simulink model "alignment_bending_procedure_n_6"  (R2018b)
settings: Solver=VariableStepAuto  StartTime=0.0  StopTime=6  RelTol=1e-3
values from neighbouring files (symbols this model uses):
  base_size = [0.2 0.3 1.5]    [robot_setup.m]    (also in robot_setup_bis.m)
  beam_length = 1.14    [robot_setup.m]    (also in robot_setup_bis.m)
  beam_radius = 0.032    [robot_setup.m]    (also in robot_setup_bis.m)
  beam_state_wf_des = fixture_keypoints(fixture_height, fixture_y, n_keypoints)    [robot_setup.m]    (also in robot_setup_bis.m)
  fixture_height = 1.5    [robot_setup.m]    (also in robot_setup_bis.m)
  fixture_x = 0.8    [robot_setup.m]    (also in robot_setup_bis.m)
  J = fscanf(fileID, '    [jacobian_mean_std.m]    (also in robot_setup.m = J_array{i-n_start+1}; robot_setup_bis.m = J_array{i-n_start+1})
  n_keypoints = i    [robot_setup.m]    (also in robot_setup_bis.m)
  robot_frame_x = 0.15    [robot_setup.m]    (also in robot_setup_bis.m)
  T = 0.005    [robot_setup.m]    (also in robot_setup_bis.m; sim_robot_control_error.m)
  wf_T_rf_left = [R_left, xyz_left'; 0 0 0 1]    [robot_setup.m]    (also in robot_setup_bis.m)
  wf_T_rf_right = [R_right, xyz_right'; 0 0 0 1]    [robot_setup.m]    (also in robot_setup_bis.m)
  xyz_0_rf_left = xyz_0_rf_left(1:3)    [robot_setup.m]    (also in robot_setup_bis.m)
  xyz_0_rf_right = xyz_0_rf_right(1:3)    [robot_setup.m]    (also in robot_setup_bis.m)
undefined symbols (not defined in the file or in its folder): beam_wall, beam_width, Extr_Data_Box, Levenberg, Marquardt, X, Y, Z
libraries: sm_lib x331, nesl_utility x53, sm_flex_body_lib x12, robotcorelib x4, simulink x2, robotmaniplib x2
(part 1 of 8)
settings Model: Creator=alberto  LastModifiedBy=alberto

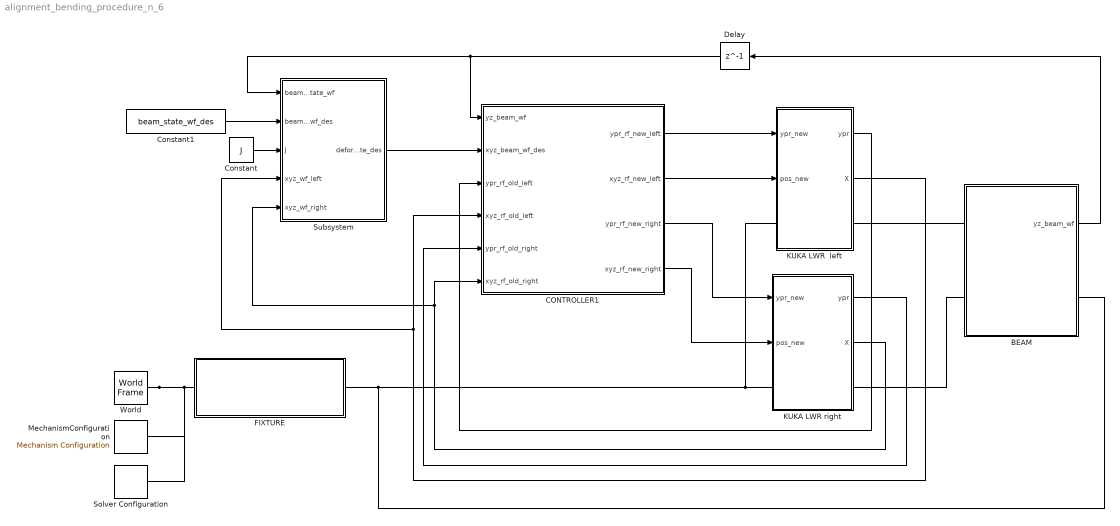
== system alignment_bending_procedure_n_6 ==
  BEAM : Subsystem
  CONTROLLER1 : Subsystem
  Constant : Constant  Value=J
  Constant1 : Constant  Value=beam_state_wf_des
  Delay : Delay  DelayLength=1  InitialCondition=-9999*ones(2*n_keypoints,1)
  FIXTURE : Subsystem
  KUKA LWR  left : Subsystem  mask{base_initial_position=[0 robot_frame_x base_size(3)-0.1]', base_initial_orientation=[pi/2 0 -pi/2]', ee_initial_position=xyz_0_rf_left, ee_initial_orientation=[0 5*pi/6 0]'}
      mask prompts: base_initial_position "base initial position [x y z]' (m)"; base_initial_orientation "base initial orientation [y p r]' (rad)"; ee_initial_position "ee initial position [x y z]' (m)"; ee_initial_orientation "ee initial orientation [y p r]' (rad)"
  KUKA LWR right : Subsystem  mask{base_initial_position=[0 -robot_frame_x base_size(3)-0.1]', base_initial_orientation=[-pi/2 0 pi/2]', ee_initial_position=xyz_0_rf_right, ee_initial_orientation=[0 5*pi/6 0]'}
      mask prompts: base_initial_position "base initial position [x y z]' (m)"; base_initial_orientation "base initial orientation [y p r]' (rad)"; ee_initial_position "ee initial position [x y z]' (m)"; ee_initial_orientation "ee initial orientation [y p r]' (rad)"
  MechanismConfiguration : sm_lib/Utilities/Mechanism Configuration  UniformGravity=Constant  GravityVector=[0 0 -9.80665]  GravityUnits=m/s^2  LinearizationDelta=0.001
  Solver Configuration : nesl_utility/Solver Configuration  PhysicalDomain=network_engine_domain  SubClassName=solver  LeftPortType=input  RightPortType=generic  Tones=[]  Harmonics=[]  SimulateNoise=off  Profile=off  UseLocalSampling=off  EnableSwitchedLinearOptims=on  FrequencyDomain=off  UseCCode=off  RelTol=0.001  AbsTol=1e-06  MinStep=1e-09  ToWorkspace=off  RevertToSquareIcSolve=off  NumHomotopyIterations=100  PhasorMode=off  PhasorModeNumHarmonics=1  DoDC=off  ResidualTolerance=1e-09  UseLocalSolver=off  LocalSolverChoice=NE_BACKWARD_EULER_ADVANCER  LocalSolverSampleTime=0.001  DoFixedCost=off  MaxNonlinIter=3  MaxModeIter=2  LinearAlgebra=auto  EquationFormulation=NE_TIME_EF  DelaysMemoryBudget=1024  AutomaticFiltering=on  FilteringTimeConstant=0.001  PartitionStorageMethod=AS_NEEDED  PartitionMemoryBudget=1024
  Subsystem : Subsystem
  World : sm_lib/Frames and Transforms/World Frame
  wires:
  KUKA LWR right/1(ypr) -> CONTROLLER1/5(ypr_rf_old_right)
  CONTROLLER1/1(ypr_rf_new_left) -> KUKA LWR  left/1(ypr_new)
  KUKA LWR  left/1(ypr) -> CONTROLLER1/3(ypr_rf_old_left)
  KUKA LWR  left/2(X) -> CONTROLLER1/4(xyz_rf_old_left), Subsystem/4(xyz_wf_left)
  CONTROLLER1/2(xyz_rf_new_left) -> KUKA LWR  left/2(pos_new)
  KUKA LWR right/2(X) -> CONTROLLER1/6(xyz_rf_old_right), Subsystem/5(xyz_wf_right)
  CONTROLLER1/4(xyz_rf_new_right) -> KUKA LWR right/2(pos_new)
  CONTROLLER1/3(ypr_rf_new_right) -> KUKA LWR right/1(ypr_new)
  Constant1/1 -> Subsystem/2(beam_state_wf_des)
  Constant/1 -> Subsystem/3(J)
  Subsystem/1(deformation_state_des) -> CONTROLLER1/2(xyz_beam_wf_des)
  Delay/1 -> CONTROLLER1/1(yz_beam_wf), Subsystem/1(beam_state_wf)
  BEAM/1("yz_beam_wf ") -> Delay/1
  connections:
  BEAM/LConn1 -- KUKA LWR  left/RConn1
  KUKA LWR  left/LConn1 -- BEAM/RConn1 -- FIXTURE/RConn1 -- KUKA LWR right/LConn1
  BEAM/LConn2 -- KUKA LWR right/RConn1
  World/RConn1 -- Solver Configuration/RConn1 -- MechanismConfiguration/RConn1 -- FIXTURE/LConn1

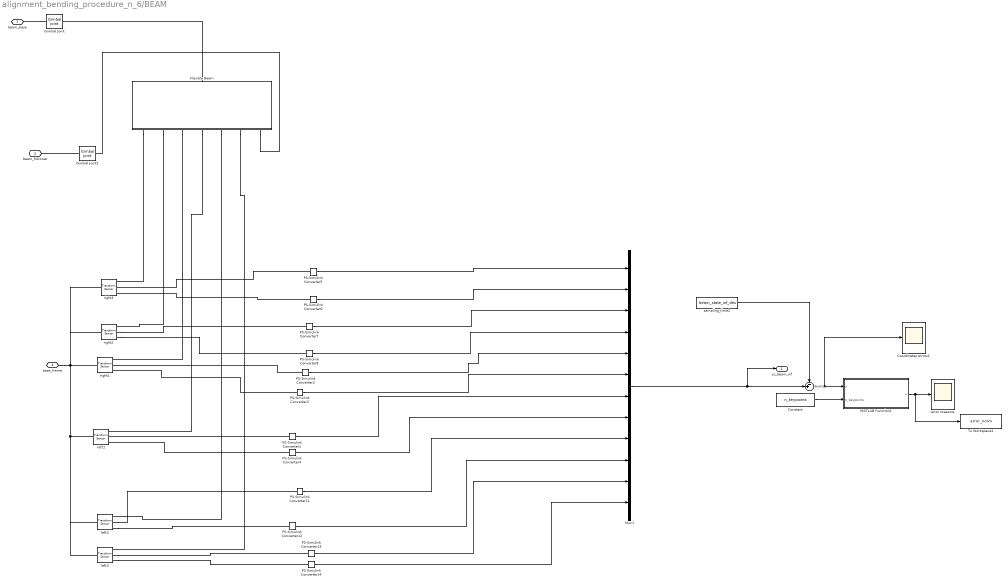
== system alignment_bending_procedure_n_6/BEAM ==
  Constant : Constant  Value=n_keypoints
  Coordinates errors1 : Scope
  Flexible Beam : Subsystem  Tag=PublishSubsystem  AncestorBlock=sm_flex_body_lib/Lumped Parameter/Bodies/Flexible Beam  mask(Flexible Body, Lumped Parameter){popup_material=Aluminum, rho_cust=975, youngsM_cust=0.8e+9, shearM_cust=0.117e+9, rho_std=2.800e+03, youngsM_std=7.000e+10, shearM_std=2.700e+10, edf_beam=2.5807e-05, sdf_beam=3.2259e-06, checkbox_internalvalues=off, popup_xc=Hollow Circle, beam_width=0.05, beam_width_in=0, beam_height=0.005, beam_height_in=0, circle_diameter=beam_radius, circle_diameter_in=0, custom_ixx=2.6121e-003, custom_iyy=2.6121e-003, custom_ip=5.2242e-003, custom_j=1.5625e-09, extrusion_data_custom=[0.015 0.005;-0.015 0.005;-0.015 -0.005;0.015 -0.005]/2, beam_length=beam_length, elem_length=0.095, numelem=12, extrusion_data=Extr_Data_Box(beam_width,beam_width-2*beam_wall,beam_width,beam_width-2*beam_wall), beam_color=[0 1 0], beam_opacity=1, radio_flextype=Rotation: Z}
      mask prompts: checkbox_internalvalues "Print internal values to Command Window"; popup_xc "Cross-Section Type"; custom_ixx "Area Ixx"; custom_iyy "Area Iyy"; custom_ip "Polar Ip"; custom_j "Torsion J (m^4)"; extrusion_data_custom "Extrusion data [x;y] (m)"; beam_length "Length (m)"; numelem "Number of elements"; beam_color "Color [RGB]"; beam_opacity "Opacity (0-1)"; radio_flextype "Flexible Element Degrees of Freedom"
      mask help: Models a flexible beam based on lumped parameter method. Number of flexible elements, material properties as well as beam cross section and dimensions can be varied from mask parameters.
      mask init:
      | cur_blk = gcb;
      | 
      | if(popup_xc==1)
      |     extrusion_data = Extr_Data_Box(beam_width,beam_width_in,beam_height,beam_height_in);
      |     xc_props = [beam_width beam_width_in beam_height beam_height_in];
      | elseif(popup_xc==2)
      |     extrusion_data = Extr_Data_Ring(circle_diameter/2,circle_diameter_in/2,0,360);
      |     xc_props = [circle_diameter circle_diameter_in];
      | elseif(popup_xc==3)
      |     extrusion_data = extrusion_data_custom;
      |     extrusion_data_vec = reshape(extrusion_data,[length(extrusion_data)*2,1]);
      |     xc_props = [custom_ixx;custom_iyy;custom_ip;custom_j;extrusion_data_vec];
      | end
      | 
      | if(popup_material == 1)
      |     rho = rho_cust;
      |     youngsM = youngsM_cust;
      |     shearM = shearM_cust;
      | else
      |     rho = rho_std;
      |     youngsM = youngsM_std;
      |     shearM = shearM_std;
      | end
      | 
      | 
      | [krot_beamz, krot_beamy, krot_beamx, ktra_beamx,...
      |     brot_beamz, brot_beamy, brot_beamx, btra_beamx, ...
      |     elem_length, Ixx, Iyy, J, crossArea] = ...
      |     sm_flex_body_lib_lpar_compute_flexprop(youngsM, shearM, numelem, beam_length, ...
      |     edf_beam, sdf_beam,popup_xc, xc_props);
      | 
      | if(checkbox_internalvalues)
      |     temp_intvaltable = table(...
      |         [Ixx;Iyy;J;crossArea;elem_length;...
      |         krot_beamz;krot_beamy;krot_beamx;ktra_beamx;...
      |         brot_beamz;brot_beamy;brot_beamx;btra_beamx],...
      |         {'m^4';'m^4';'m^4';'m^2';'m';...
      |         'N*m/rad';'N*m/rad';'N*m/rad';'N/m';...
      |         'N*m/(rad/s)';'N*m/(rad/s)';'N*m/(rad/s)';'N/(m/s)'},...
      |         'VariableNames',{'Value','Units'},'RowNames',...
      |         {'Area Moment of Inertia, Ixx','Area Moment of Inertia, Iyy',...
      |         'Torsional Constant, J','Cross sectional area, A','Flexible element length',...
      |         'Element Stiffness, Bending about Z','Element Stiffness, Bending about Y',...
      |         'Element Stiffness, Torsion about X','Element Stiffness, Elongation along X',...
      |         'Element Damping, Bending about Z','Element Damping, Bending about Y',...
      |         'Element Damping, Torsion about X','Element Damping, Elongation along X'});
      |     disp(temp_intvaltable);
      | end
      | 
      | set_param(cur_blk,'elem_length',num2str(elem_length));
      | 
      | sm_flex_body_lib_lpar_construct_beam(cur_blk,numelem,get_param(cur_blk,'radio_flextype'));
      | 
      | clear xc_props
      settings: CopyFcn=%set_param(gcb, 'LinkStatus', 'none')
      settings: AttributesFormatString=|
      | No of Elem: 12
      | Rotation: Z
      mask Help: web('sm_flex_body_lib_lumped_par_beam.html')
      mask TypeOptions popup_material: Custom | Steel | Aluminum | Brass | Bismuth | Copper | Gold | Iron | Lead | Magnesium | Nickel | Silver | Tin | Zinc
      mask Callback popup_material:
      | maskObj = Simulink.Mask.get(gcb);
      | contcm_h = maskObj.getDialogControl('cont_custmaterial');
      | contsm_h = maskObj.getDialogControl('cont_stdmaterial');
      | 
      | rhostd_h = maskObj.getParameter('rho_std');
      | youngM_h = maskObj.getParameter('youngsM_std');
      | shearM_h = maskObj.getParameter('shearM_std');
      | 
      | popup_cm = get_param(gcb,'popup_material');
      | if strcmp(popup_cm,'Custom')
      |     contcm_h.Visible = 'on';
      |     contsm_h.Visible = 'off';
      | else
      |     [rho, E, G] = sm_flex_body_lib_lpar_matprops(popup_cm);
      |     rhostd_h.ReadOnly = 'off';
      |     youngM_h.ReadOnly = 'off';
      |     shearM_h.ReadOnly = 'off';
      |     set_param(gcb,'rho_std',sprintf('%0.3e',rho));
      |     set_param(gcb,'youngsM_std',sprintf('%0.3e',E));
      |     set_param(gcb,'shearM_std',sprintf('%0.3e',G));
      | 	rhostd_h.ReadOnly = 'on';
      |     youngM_h.ReadOnly = 'on';
      |     shearM_h.ReadOnly = 'on';
      |     contcm_h.Visible = 'off';
      |     contsm_h.Visible = 'on';
      | end
      | 
      | clear maskObj contcm_h contsm_h
      | clear rhostd_h youngM_h shearM_h rho E G
      mask TypeOptions popup_xc: Hollow Rectangle | Hollow Circle | Custom
      mask Callback popup_xc:
      | maskObj = Simulink.Mask.get(gcb);
      | rcti_h = maskObj.getDialogControl('container_rectimage');
      | rctp_h = maskObj.getDialogControl('container_rectparams');
      | ciri_h = maskObj.getDialogControl('container_circleimage');
      | cirp_h = maskObj.getDialogControl('container_circleparams');
      | cusi_h = maskObj.getDialogControl('container_customimage');
      | cusp_h = maskObj.getDialogControl('container_customparams');
      | 
      | popd_h = maskObj.getParameter('popup_dampparam');
      | contdr_h = maskObj.getDialogControl('cont_dampingratio');
      | contdc_h = maskObj.getDialogControl('cont_dampingcoeff');
      | 
      | rcti_h.Visible = 'off';
      | rctp_h.Visible = 'off';
      | ciri_h.Visible = 'off';
      | cirp_h.Visible = 'off';
      | cusi_h.Visible = 'off';
      | cusp_h.Visible = 'off';
      | 
      | if strcmp(get_param(gcb,'popup_xc'),'Hollow Rectangle')
      |     rcti_h.Visible = 'on';
      |     rctp_h.Visible = 'on';
      | elseif strcmp(get_param(gcb,'popup_xc'),'Hollow Circle')
      |     ciri_h.Visible = 'on';
      |     cirp_h.Visible = 'on';
      | elseif strcmp(get_param(gcb,'popup_xc'),'Custom')
      |     cusi_h.Visible = 'on';
      |     cusp_h.Visible = 'on';
      | end
      | 
      | clear rcti_h rctp_h ciri_h cirp_h cusi_h cusp_h
      mask TypeOptions radio_flextype: Rotation: Z | Rotation: X, Y, Z; Translation: X
      mask DialogControl tab_material Prompt: Material
      mask DialogControl Control20 Prompt: Material
      mask DialogControl Control22 Prompt: Material Density (kg/(m^3))
      mask DialogControl Control23 Prompt: Modulus of Elasticity (N/m^2)
      mask DialogControl Control24 Prompt: Shear Modulus (N/m^2)
      mask DialogControl grp_damping Prompt: Damping
      mask DialogControl Control26 Prompt: Elastic Damping Factor (sec)
      mask DialogControl Control27 Prompt: Shear Damping Factor (sec)
      mask DialogControl tab_geometry Prompt: Geometry
      mask DialogControl text_outer Prompt: Outer
      mask DialogControl text_inner Prompt: Inner
      mask DialogControl text_width Prompt: Width (m)
      mask DialogControl text_height Prompt: Height (m)
      mask DialogControl text_circle_outer Prompt: Outer
      mask DialogControl text_circle_inner Prompt: Inner
      mask DialogControl text_circle_width Prompt: Diameter (m)
      mask DialogControl cont_custmoi Prompt: Moment of Inertia (m^4)
      mask DialogControl tab_flextype Prompt: Flexibility Type
      mask Display: image('sm_flex_body_lib_lumpparbeam_IMAGE.png');
  Gimbal Joint : sm_lib/Joints/Gimbal Joint  SenseConstraintForce=off  SenseConstraintForceX=off  SenseConstraintForceY=off  SenseConstraintForceZ=off  SenseConstraintTorque=off  SenseConstraintTorqueX=off  SenseConstraintTorqueY=off  SenseConstraintTorqueZ=off  SenseTotalForce=off  SenseTotalForceX=off  SenseTotalForceY=off  SenseTotalForceZ=off  SenseTotalTorque=off  SenseTotalTorqueX=off  SenseTotalTorqueY=off  SenseTotalTorqueZ=off  CompositeWrenchDir=FollowerOnBase  CompositeWrenchFrame=BaseFrame  RxEquilibriumPosition=0  RxEquilibriumPositionUnits=deg  RxSpringStiffness=0  RxSpringStiffnessUnits=N*m/deg  RxDampingCoefficient=0  RxDampingCoefficientUnits=N*m/(deg/s)  RxTorqueActuationMode=NoTorque  RxMotionActuationMode=ComputedMotion  RxSensePosition=off  RxSenseVelocity=off  RxSenseAcceleration=off  RxSenseTorqueForce=off  RxPositionTargetSpecify=off  RxPositionTargetPriority=High  RxPositionTargetValue=0  RxPositionTargetValueUnits=deg  RxVelocityTargetSpecify=off  RxVelocityTargetPriority=High  RxVelocityTargetValue=0  RxVelocityTargetValueUnits=deg/s  RyEquilibriumPosition=0  RyEquilibriumPositionUnits=deg  RySpringStiffness=2000  RySpringStiffnessUnits=N*m/deg  RyDampingCoefficient=1  RyDampingCoefficientUnits=N*m/(deg/s)  RyTorqueActuationMode=NoTorque  RyMotionActuationMode=ComputedMotion  RySensePosition=off  RySenseVelocity=off  RySenseAcceleration=off  RySenseTorqueForce=off  RyPositionTargetSpecify=off  RyPositionTargetPriority=High  RyPositionTargetValue=0  RyPositionTargetValueUnits=deg  RyVelocityTargetSpecify=off  RyVelocityTargetPriority=High  RyVelocityTargetValue=0  RyVelocityTargetValueUnits=deg/s  RzEquilibriumPosition=0  RzEquilibriumPositionUnits=deg  RzSpringStiffness=0  RzSpringStiffnessUnits=N*m/deg  RzDampingCoefficient=0  RzDampingCoefficientUnits=N*m/(deg/s)  RzTorqueActuationMode=NoTorque  RzMotionActuationMode=ComputedMotion  RzSensePosition=off  RzSenseVelocity=off  RzSenseAcceleration=off  RzSenseTorqueForce=off  RzPositionTargetSpecify=off  RzPositionTargetPriority=High  RzPositionTargetValue=0  RzPositionTargetValueUnits=deg  RzVelocityTargetSpecify=off  RzVelocityTargetPriority=High  RzVelocityTargetValue=0  RzVelocityTargetValueUnits=deg/s
      settings: SourceProductName=Simscape Multibody
  Gimbal Joint1 : sm_lib/Joints/Gimbal Joint  SenseConstraintForce=off  SenseConstraintForceX=off  SenseConstraintForceY=off  SenseConstraintForceZ=off  SenseConstraintTorque=off  SenseConstraintTorqueX=off  SenseConstraintTorqueY=off  SenseConstraintTorqueZ=off  SenseTotalForce=off  SenseTotalForceX=off  SenseTotalForceY=off  SenseTotalForceZ=off  SenseTotalTorque=off  SenseTotalTorqueX=off  SenseTotalTorqueY=off  SenseTotalTorqueZ=off  CompositeWrenchDir=FollowerOnBase  CompositeWrenchFrame=BaseFrame  RxEquilibriumPosition=0  RxEquilibriumPositionUnits=deg  RxSpringStiffness=0  RxSpringStiffnessUnits=N*m/deg  RxDampingCoefficient=0  RxDampingCoefficientUnits=N*m/(deg/s)  RxTorqueActuationMode=NoTorque  RxMotionActuationMode=ComputedMotion  RxSensePosition=off  RxSenseVelocity=off  RxSenseAcceleration=off  RxSenseTorqueForce=off  RxPositionTargetSpecify=off  RxPositionTargetPriority=High  RxPositionTargetValue=0  RxPositionTargetValueUnits=deg  RxVelocityTargetSpecify=off  RxVelocityTargetPriority=High  RxVelocityTargetValue=0  RxVelocityTargetValueUnits=deg/s  RyEquilibriumPosition=0  RyEquilibriumPositionUnits=deg  RySpringStiffness=2000  RySpringStiffnessUnits=N*m/deg  RyDampingCoefficient=1  RyDampingCoefficientUnits=N*m/(deg/s)  RyTorqueActuationMode=NoTorque  RyMotionActuationMode=ComputedMotion  RySensePosition=off  RySenseVelocity=off  RySenseAcceleration=off  RySenseTorqueForce=off  RyPositionTargetSpecify=off  RyPositionTargetPriority=High  RyPositionTargetValue=0  RyPositionTargetValueUnits=deg  RyVelocityTargetSpecify=off  RyVelocityTargetPriority=High  RyVelocityTargetValue=0  RyVelocityTargetValueUnits=deg/s  RzEquilibriumPosition=0  RzEquilibriumPositionUnits=deg  RzSpringStiffness=0  RzSpringStiffnessUnits=N*m/deg  RzDampingCoefficient=0  RzDampingCoefficientUnits=N*m/(deg/s)  RzTorqueActuationMode=NoTorque  RzMotionActuationMode=ComputedMotion  RzSensePosition=off  RzSenseVelocity=off  RzSenseAcceleration=off  RzSenseTorqueForce=off  RzPositionTargetSpecify=off  RzPositionTargetPriority=High  RzPositionTargetValue=0  RzPositionTargetValueUnits=deg  RzVelocityTargetSpecify=off  RzVelocityTargetPriority=High  RzVelocityTargetValue=0  RzVelocityTargetValueUnits=deg/s
      settings: SourceProductName=Simscape Multibody
  MATLAB Function1 : MATLAB Function  TreatAsAtomicUnit=on
  Mux1 : Mux  Inputs=12
  PS-Simulink Converter{1..8,11..14} (12 alike) : nesl_utility/PS-Simulink Converter  PhysicalDomain=network_engine_domain  SubClassName=ps_output  LeftPortType=input  RightPortType=output  PseudoPeriodic=off  Frequencies=[]  Unit=1  AffineConversion=off
  Sum1 : Sum  Inputs=-+|
  To Workspace1 : ToWorkspace  VariableName=error_norm  SampleTime=T
      settings: Save2DSignal=2-D array (concatenate along first dimension)
  error measure : Scope
  left1 : sm_lib/Frames and Transforms/Transform Sensor  MeasurementFrame=Base  SenseAngle=off  SenseAxis=off  SenseAngle1=off  SenseAngle2=off  SenseAngle3=off  SenseQ=off  SenseR=off  SenseOmegaX=off  SenseOmegaY=off  SenseOmegaZ=off  SenseOmega1=off  SenseOmega2=off  SenseOmega3=off  SenseQDot=off  SenseRDot=off  SenseAlphaX=off  SenseAlphaY=off  SenseAlphaZ=off  SenseAlpha1=off  SenseAlpha2=off  SenseAlpha3=off  SenseQDDot=off  SenseRDDot=off  SenseX=off  SenseY=on  SenseZ=on  SenseRad=off  SenseAzim=off  SenseDist=off  SenseInc=off  SenseXDot=off  SenseYDot=off  SenseZDot=off  SenseRadDot=off  SenseAzimDot=off  SenseDistDot=off  SenseIncDot=off  SenseXDDot=off  SenseYDDot=off  SenseZDDot=off  SenseRadDDot=off  SenseAzimDDot=off  SenseDistDDot=off  SenseIncDDot=off
  left2 : sm_lib/Frames and Transforms/Transform Sensor  MeasurementFrame=Base  SenseAngle=off  SenseAxis=off  SenseAngle1=off  SenseAngle2=off  SenseAngle3=off  SenseQ=off  SenseR=off  SenseOmegaX=off  SenseOmegaY=off  SenseOmegaZ=off  SenseOmega1=off  SenseOmega2=off  SenseOmega3=off  SenseQDot=off  SenseRDot=off  SenseAlphaX=off  SenseAlphaY=off  SenseAlphaZ=off  SenseAlpha1=off  SenseAlpha2=off  SenseAlpha3=off  SenseQDDot=off  SenseRDDot=off  SenseX=off  SenseY=on  SenseZ=on  SenseRad=off  SenseAzim=off  SenseDist=off  SenseInc=off  SenseXDot=off  SenseYDot=off  SenseZDot=off  SenseRadDot=off  SenseAzimDot=off  SenseDistDot=off  SenseIncDot=off  SenseXDDot=off  SenseYDDot=off  SenseZDDot=off  SenseRadDDot=off  SenseAzimDDot=off  SenseDistDDot=off  SenseIncDDot=off
  left3 : sm_lib/Frames and Transforms/Transform Sensor  MeasurementFrame=Base  SenseAngle=off  SenseAxis=off  SenseAngle1=off  SenseAngle2=off  SenseAngle3=off  SenseQ=off  SenseR=off  SenseOmegaX=off  SenseOmegaY=off  SenseOmegaZ=off  SenseOmega1=off  SenseOmega2=off  SenseOmega3=off  SenseQDot=off  SenseRDot=off  SenseAlphaX=off  SenseAlphaY=off  SenseAlphaZ=off  SenseAlpha1=off  SenseAlpha2=off  SenseAlpha3=off  SenseQDDot=off  SenseRDDot=off  SenseX=off  SenseY=on  SenseZ=on  SenseRad=off  SenseAzim=off  SenseDist=off  SenseInc=off  SenseXDot=off  SenseYDot=off  SenseZDot=off  SenseRadDot=off  SenseAzimDot=off  SenseDistDot=off  SenseIncDot=off  SenseXDDot=off  SenseYDDot=off  SenseZDDot=off  SenseRadDDot=off  SenseAzimDDot=off  SenseDistDDot=off  SenseIncDDot=off
  right1 : sm_lib/Frames and Transforms/Transform Sensor  MeasurementFrame=Base  SenseAngle=off  SenseAxis=off  SenseAngle1=off  SenseAngle2=off  SenseAngle3=off  SenseQ=off  SenseR=off  SenseOmegaX=off  SenseOmegaY=off  SenseOmegaZ=off  SenseOmega1=off  SenseOmega2=off  SenseOmega3=off  SenseQDot=off  SenseRDot=off  SenseAlphaX=off  SenseAlphaY=off  SenseAlphaZ=off  SenseAlpha1=off  SenseAlpha2=off  SenseAlpha3=off  SenseQDDot=off  SenseRDDot=off  SenseX=off  SenseY=on  SenseZ=on  SenseRad=off  SenseAzim=off  SenseDist=off  SenseInc=off  SenseXDot=off  SenseYDot=off  SenseZDot=off  SenseRadDot=off  SenseAzimDot=off  SenseDistDot=off  SenseIncDot=off  SenseXDDot=off  SenseYDDot=off  SenseZDDot=off  SenseRadDDot=off  SenseAzimDDot=off  SenseDistDDot=off  SenseIncDDot=off
  right2 : sm_lib/Frames and Transforms/Transform Sensor  MeasurementFrame=Base  SenseAngle=off  SenseAxis=off  SenseAngle1=off  SenseAngle2=off  SenseAngle3=off  SenseQ=off  SenseR=off  SenseOmegaX=off  SenseOmegaY=off  SenseOmegaZ=off  SenseOmega1=off  SenseOmega2=off  SenseOmega3=off  SenseQDot=off  SenseRDot=off  SenseAlphaX=off  SenseAlphaY=off  SenseAlphaZ=off  SenseAlpha1=off  SenseAlpha2=off  SenseAlpha3=off  SenseQDDot=off  SenseRDDot=off  SenseX=off  SenseY=on  SenseZ=on  SenseRad=off  SenseAzim=off  SenseDist=off  SenseInc=off  SenseXDot=off  SenseYDot=off  SenseZDot=off  SenseRadDot=off  SenseAzimDot=off  SenseDistDot=off  SenseIncDot=off  SenseXDDot=off  SenseYDDot=off  SenseZDDot=off  SenseRadDDot=off  SenseAzimDDot=off  SenseDistDDot=off  SenseIncDDot=off
  right3 : sm_lib/Frames and Transforms/Transform Sensor  MeasurementFrame=Base  SenseAngle=off  SenseAxis=off  SenseAngle1=off  SenseAngle2=off  SenseAngle3=off  SenseQ=off  SenseR=off  SenseOmegaX=off  SenseOmegaY=off  SenseOmegaZ=off  SenseOmega1=off  SenseOmega2=off  SenseOmega3=off  SenseQDot=off  SenseRDot=off  SenseAlphaX=off  SenseAlphaY=off  SenseAlphaZ=off  SenseAlpha1=off  SenseAlpha2=off  SenseAlpha3=off  SenseQDDot=off  SenseRDDot=off  SenseX=off  SenseY=on  SenseZ=on  SenseRad=off  SenseAzim=off  SenseDist=off  SenseInc=off  SenseXDot=off  SenseYDot=off  SenseZDot=off  SenseRadDot=off  SenseAzimDot=off  SenseDistDot=off  SenseIncDot=off  SenseXDDot=off  SenseYDDot=off  SenseZDDot=off  SenseRadDDot=off  SenseAzimDDot=off  SenseDistDDot=off  SenseIncDDot=off
  sampling_time2 : Constant  Value=beam_state_wf_des
  beam_base : PMIOPort  Side=Left
  beam_follower : PMIOPort  Port=2  Side=Left
  base_frame : PMIOPort  Port=3  Side=Right
  "yz_beam_wf " : Outport
  wires:
  PS-Simulink Converter5/1 -> Mux1/1
  PS-Simulink Converter6/1 -> Mux1/2
  PS-Simulink Converter7/1 -> Mux1/3
  PS-Simulink Converter8/1 -> Mux1/4
  PS-Simulink Converter2/1 -> Mux1/5
  PS-Simulink Converter3/1 -> Mux1/6
  PS-Simulink Converter1/1 -> Mux1/7
  PS-Simulink Converter4/1 -> Mux1/8
  PS-Simulink Converter11/1 -> Mux1/9
  PS-Simulink Converter12/1 -> Mux1/10
  PS-Simulink Converter13/1 -> Mux1/11
  PS-Simulink Converter14/1 -> Mux1/12
  Mux1/1 -> "yz_beam_wf "/1, Sum1/2
  Constant/1 -> MATLAB Function1/2(n_keypoints)
  MATLAB Function1/1(y) -> To Workspace1/1, error measure/1
  sampling_time2/1 -> Sum1/1
  Sum1/1 -> Coordinates errors1/1, MATLAB Function1/1(u)
  connections:
  base_frame/RConn1 -- left1/LConn1 -- left3/LConn1 -- left2/LConn1 -- right1/LConn1 -- right3/LConn1 -- right2/LConn1
  PS-Simulink Converter3/LConn1 -- right1/RConn3
  PS-Simulink Converter5/LConn1 -- right3/RConn2
  PS-Simulink Converter4/LConn1 -- left1/RConn3
  PS-Simulink Converter2/LConn1 -- right1/RConn2
  Gimbal Joint/LConn1 -- beam_base/RConn1
  PS-Simulink Converter6/LConn1 -- right3/RConn3
  Flexible Beam/RConn1 -- Gimbal Joint1/RConn1
  right2/RConn2 -- PS-Simulink Converter7/LConn1
  right2/RConn3 -- PS-Simulink Converter8/LConn1
  Flexible Beam/LConn1 -- Gimbal Joint/RConn1
  PS-Simulink Converter1/LConn1 -- left1/RConn2
  Gimbal Joint1/LConn1 -- beam_follower/RConn1
  left2/RConn2 -- PS-Simulink Converter11/LConn1
  left2/RConn3 -- PS-Simulink Converter12/LConn1
  left3/RConn2 -- PS-Simulink Converter13/LConn1
  left3/RConn3 -- PS-Simulink Converter14/LConn1
  Flexible Beam/RConn7 -- right3/RConn1
  Flexible Beam/RConn6 -- right2/RConn1
  Flexible Beam/RConn5 -- right1/RConn1
  Flexible Beam/RConn4 -- left1/RConn1
  Flexible Beam/RConn3 -- left2/RConn1
  Flexible Beam/RConn2 -- left3/RConn1

== system alignment_bending_procedure_n_6/CONTROLLER1 ==
  yz_beam_wf : Inport
  xyz_beam_wf_des : Inport  Port=2
  ypr_rf_old_left : Inport  Port=3
  xyz_rf_old_left : Inport  Port=4
  ypr_rf_old_right : Inport  Port=5
  xyz_rf_old_right : Inport  Port=6
  CONTROLLER : Subsystem
  ypr_rf_new_left : Outport
  xyz_rf_new_left : Outport  Port=2
  ypr_rf_new_right : Outport  Port=3
  xyz_rf_new_right : Outport  Port=4
  wires:
  CONTROLLER/1(ypr_rf_new_left) -> ypr_rf_new_left/1
  CONTROLLER/2(ypr_rf_new_right) -> ypr_rf_new_right/1
  ypr_rf_old_right/1 -> CONTROLLER/6(ypr_rf_old_right)
  ypr_rf_old_left/1 -> CONTROLLER/5(ypr_rf_old_left)
  xyz_rf_old_left/1 -> CONTROLLER/3("xyz_rf_old_left ")
  xyz_rf_old_right/1 -> CONTROLLER/4(xyz_rf_old_right)
  xyz_beam_wf_des/1 -> CONTROLLER/2(xyz_beam_wf_des)
  CONTROLLER/3(xyz_rf_new_left) -> xyz_rf_new_left/1
  CONTROLLER/4(xyz_rf_new_right) -> xyz_rf_new_right/1
  yz_beam_wf/1 -> CONTROLLER/1(xyz_beam_wf_old)

== system alignment_bending_procedure_n_6/FIXTURE ==
  FIXTURE : Subsystem
  Reference Frame : sm_lib/Frames and Transforms/Reference Frame
  Rigid Transform : sm_lib/Frames and Transforms/Rigid Transform  TranslationMethod=Cartesian  TranslationStandardOffset=0  TranslationLengthUnit=m  TranslationStandardAxis=+Z  TranslationCartesianOffset=[0 0 base_size(3)/2]  TranslationROffset=0  TranslationROffsetUnits=m  TranslationZOffset=0  TranslationZOffsetUnits=m  TranslationThetaOffset=0  TranslationThetaOffsetUnits=deg  RotationMethod=None  RotationAngleUnits=deg  RotationStandardAxis=+Z  RotationAngle=0.0  RotationArbitraryAxis=[0 0 1]  FollAlignAxisA=+X  BaseAlignAxisA=+Y  FollAlignAxisB=+Y  BaseAlignAxisB=+Z  RotationSequenceAxes=FollowerAxes  RotationSequence=XYX  RotationSequenceAngles=[0 0 0]  RotationSequenceAnglesUnits=deg  RotationMatrix=[1 0 0; 0 1 0; 0 0 1]
  Rigid Transform1 : sm_lib/Frames and Transforms/Rigid Transform  TranslationMethod=Cartesian  TranslationStandardOffset=0  TranslationLengthUnit=m  TranslationStandardAxis=+Z  TranslationCartesianOffset=[0 0 -base_size(3)/2]  TranslationROffset=0  TranslationROffsetUnits=m  TranslationZOffset=0  TranslationZOffsetUnits=m  TranslationThetaOffset=0  TranslationThetaOffsetUnits=deg  RotationMethod=None  RotationAngleUnits=deg  RotationStandardAxis=+Z  RotationAngle=0.0  RotationArbitraryAxis=[0 0 1]  FollAlignAxisA=+X  BaseAlignAxisA=+Y  FollAlignAxisB=+Y  BaseAlignAxisB=+Z  RotationSequenceAxes=FollowerAxes  RotationSequence=XYX  RotationSequenceAngles=[0 0 0]  RotationSequenceAnglesUnits=deg  RotationMatrix=[1 0 0; 0 1 0; 0 0 1]
  Solid : sm_lib/Body Elements/Solid  InertiaType=CalculateFromGeometry  Mass=1  MassUnits=kg  CenterOfMass=[0 0 0]  CenterOfMassUnits=m  MomentsOfInertia=[1 1 1]  MomentsOfInertiaUnits=kg*m^2  ProductsOfInertia=[0 0 0]  ProductsOfInertiaUnits=kg*m^2  BasedOnType=Density  Density=1000  DensityUnits=kg/m^3  DoExposeReferenceFrame=on  SerializedFrames=<Frames/>  GraphicType=FromGeometry  MarkerShape=Sphere  MarkerSize=10  GraphicVisPropType=SimpleVisualProperties  GraphicDiffuseColor=[0.0 0.0 0.8]  GraphicSpecularColor=[0.5 0.5 0.5 1.0]  GraphicAmbientColor=[0.15 0.15 0.15 1.0]  GraphicEmissiveColor=[0.0 0.0 0.0 1.0]  GraphicShininess=75  GraphicOpacity=1.0  GeometryShape=Brick  RectangleSize=[1 1]  RectangleSizeUnits=m  BrickDimensions=base_size  BrickDimensionUnits=m  CylinderRadius=1  CylinderRadiusUnits=m  CylinderLength=1  CylinderLengthUnits=m  SphereRadius=1  SphereRadiusUnits=m  EllipsoidRadii=[1 1 1]  EllipsoidRadiiUnits=m  ExtrusionCrossSection=[1 1; -1 1; -1 -1; 1 -1]  ExtrusionCrossSectionUnits=m  ExtrusionLength=1  ExtrusionLengthUnits=m  PolygonNumSides=3  PolygonOuterRadius=1  PolygonOuterRadiusUnits=m  ExtGeomFileType=STEP  ExtGeomFileUnits=m  RevolutionCrossSection=[1 1; 1 -1; 2 -1; 2 1]  RevolutionCrossSectionUnits=m  RevolutionExtent=Full  RevolutionAngle=180  RevolutionAngleUnits=deg
  dual_arm_center : PMIOPort  Side=Left
  dual_arm_bottom : PMIOPort  Port=2  Side=Right
  connections:
  Rigid Transform/LConn1 -- Solid/RConn1 -- Rigid Transform1/LConn1 -- dual_arm_center/RConn1
  dual_arm_bottom/RConn1 -- Rigid Transform1/RConn1 -- FIXTURE/LConn1
  Reference Frame/RConn1 -- Rigid Transform/RConn1

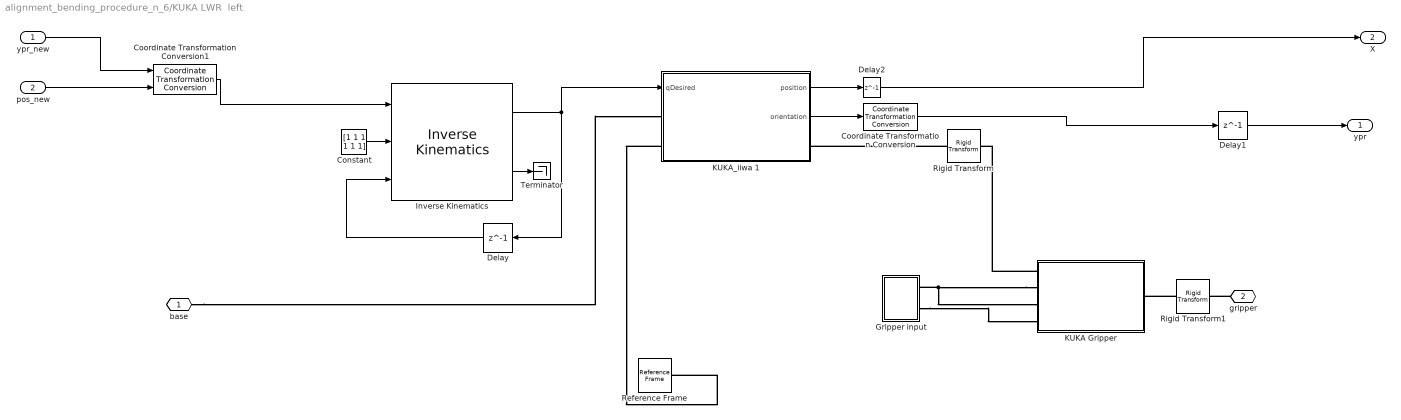
== system alignment_bending_procedure_n_6/KUKA LWR  left ==
  ypr_new : Inport
  pos_new : Inport  Port=2
  Constant : Constant  Value=[1 1 1 1 1 1]
  Coordinate Transformation Conversion : robotcorelib/Coordinate Transformation Conversion  InputRepresentation=Rotation Matrix  InputEulerSequence=ZYX  ShowTrVecInputPort=on  OutputRepresentation=Euler Angles  OutputEulerSequence=ZYX  ShowTrVecOutputPort=on  SimulateUsing=Interpreted execution
      settings: SourceProductBaseCode=RO
  Coordinate Transformation Conversion1 : robotcorelib/Coordinate Transformation Conversion  InputRepresentation=Euler Angles  InputEulerSequence=ZYX  ShowTrVecInputPort=on  OutputRepresentation=Homogeneous Transformation  OutputEulerSequence=ZYX  ShowTrVecOutputPort=on  SimulateUsing=Interpreted execution
      settings: SourceProductBaseCode=RO
  Delay : Delay  DelayLength=1  InitialCondition=[0 0 0 0 0 0 0]'  SampleTime=T
  Delay1 : Delay  DelayLength=1  InitialCondition=ee_initial_orientation
  Delay2 : Delay  DelayLength=1  InitialCondition=ee_initial_position
  Gripper input : Subsystem
  Inverse Kinematics : robotmaniplib/Inverse Kinematics  RigidBodyTree=lbr  EndEffector=iiwa_link_ee  ShowInfo=on  SolverName=Levenberg-Marquardt  EnforceJointLimits=on  MaxIterations=1500  MaxTime=10  GradientTolerance=1e-7  SolutionTolerance=1e-6  StepTolerance=1e-14  ErrorChangeTolerance=1e-12  UseErrorDamping=on  DampingBias=0.0025
      settings: SourceProductName=Robotics System Toolbox
  KUKA Gripper : Subsystem
  "KUKA_iiwa 1 " : Subsystem  mask{base_pos=base_initial_position, base_rot=base_initial_orientation}
      mask prompts: base_pos "position [x y z]' (m)"; base_rot "orientation [y p r]' (rad)"
  Reference Frame : sm_lib/Frames and Transforms/Reference Frame
  Rigid Transform : sm_lib/Frames and Transforms/Rigid Transform  TranslationMethod=None  TranslationStandardOffset=0  TranslationLengthUnit=m  TranslationStandardAxis=+Z  TranslationCartesianOffset=[0 0 0]  TranslationROffset=0  TranslationROffsetUnits=m  TranslationZOffset=0  TranslationZOffsetUnits=m  TranslationThetaOffset=0  TranslationThetaOffsetUnits=deg  RotationMethod=RotationSequence  RotationAngleUnits=deg  RotationStandardAxis=+Z  RotationAngle=0.0  RotationArbitraryAxis=[0 0 1]  FollAlignAxisA=+X  BaseAlignAxisA=+Y  FollAlignAxisB=+Y  BaseAlignAxisB=+Z  RotationSequenceAxes=FollowerAxes  RotationSequence=XYZ  RotationSequenceAngles=[-90 -90 0]  RotationSequenceAnglesUnits=deg  RotationMatrix=[1 0 0; 0 1 0; 0 0 1]
  Rigid Transform1 : sm_lib/Frames and Transforms/Rigid Transform  TranslationMethod=Cartesian  TranslationStandardOffset=0  TranslationLengthUnit=cm  TranslationStandardAxis=+Z  TranslationCartesianOffset=[2*beam_radius 0 0]  TranslationROffset=0  TranslationROffsetUnits=m  TranslationZOffset=0  TranslationZOffsetUnits=m  TranslationThetaOffset=0  TranslationThetaOffsetUnits=deg  RotationMethod=RotationSequence  RotationAngleUnits=deg  RotationStandardAxis=+Z  RotationAngle=0.0  RotationArbitraryAxis=[0 0 1]  FollAlignAxisA=+X  BaseAlignAxisA=+Y  FollAlignAxisB=+Y  BaseAlignAxisB=+Z  RotationSequenceAxes=FollowerAxes  RotationSequence=XYZ  RotationSequenceAngles=[0 0 0]  RotationSequenceAnglesUnits=deg  RotationMatrix=[1 0 0; 0 1 0; 0 0 1]
  Terminator : Terminator
  base : PMIOPort  Side=Left
  gripper : PMIOPort  Port=2  Side=Right
  ypr : Outport
  X : Outport  Port=2
  wires:
  Inverse Kinematics/1 -> "KUKA_iiwa 1 "/1(qDesired), Delay/1
  Coordinate Transformation Conversion1/1 -> Inverse Kinematics/1
  Constant/1 -> Inverse Kinematics/2
  Inverse Kinematics/2 -> Terminator/1
  "KUKA_iiwa 1 "/1(position) -> Delay2/1
  "KUKA_iiwa 1 "/2(orientation) -> Coordinate Transformation Conversion/1
  Coordinate Transformation Conversion/1 -> Delay1/1
  ypr_new/1 -> Coordinate Transformation Conversion1/1
  pos_new/1 -> Coordinate Transformation Conversion1/2
  Delay2/1 -> X/1
  Delay1/1 -> ypr/1
  Delay/1 -> Inverse Kinematics/3
  connections:
  base/RConn1 -- "KUKA_iiwa 1 "/LConn1
  KUKA Gripper/LConn1 -- Rigid Transform/RConn1
  Rigid Transform/LConn1 -- "KUKA_iiwa 1 "/RConn1
  gripper/RConn1 -- Rigid Transform1/RConn1
  Rigid Transform1/LConn1 -- KUKA Gripper/RConn1
  KUKA Gripper/LConn2 -- Gripper input/RConn1 -- KUKA Gripper/LConn3
  Gripper input/RConn2 -- KUKA Gripper/LConn4
  "KUKA_iiwa 1 "/LConn2 -- Reference Frame/RConn1

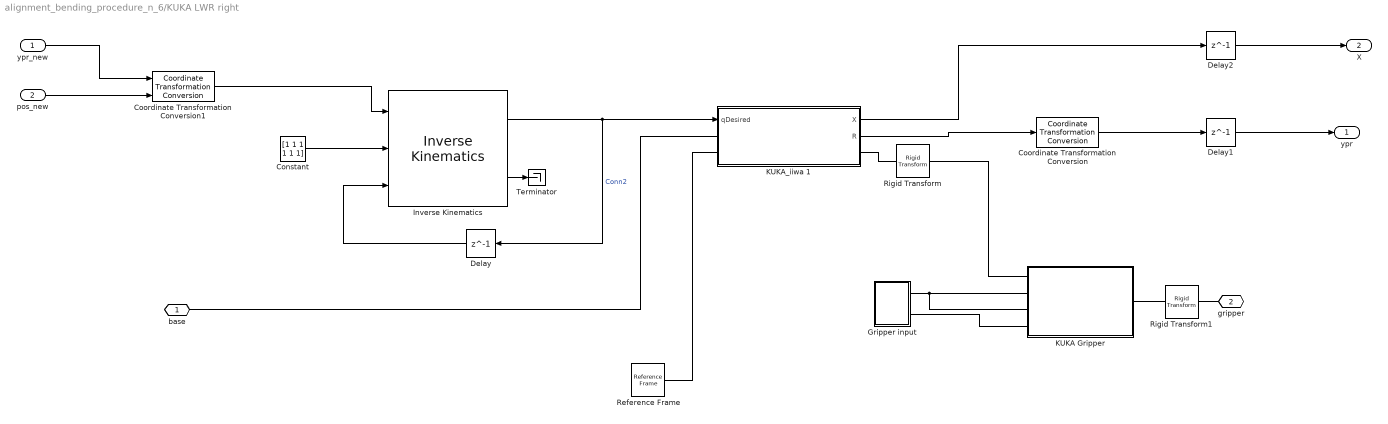
== system alignment_bending_procedure_n_6/KUKA LWR right ==
  ypr_new : Inport
  pos_new : Inport  Port=2
  Constant : Constant  Value=[1 1 1 1 1 1]
  Coordinate Transformation Conversion : robotcorelib/Coordinate Transformation Conversion  InputRepresentation=Rotation Matrix  InputEulerSequence=ZYX  ShowTrVecInputPort=on  OutputRepresentation=Euler Angles  OutputEulerSequence=ZYX  ShowTrVecOutputPort=on  SimulateUsing=Interpreted execution
      settings: SourceProductBaseCode=RO
  Coordinate Transformation Conversion1 : robotcorelib/Coordinate Transformation Conversion  InputRepresentation=Euler Angles  InputEulerSequence=ZYX  ShowTrVecInputPort=on  OutputRepresentation=Homogeneous Transformation  OutputEulerSequence=ZYX  ShowTrVecOutputPort=on  SimulateUsing=Interpreted execution
      settings: SourceProductBaseCode=RO
  Delay : Delay  DelayLength=1  InitialCondition=[0 0 0 0 0 0 0]'  SampleTime=T
  Delay1 : Delay  DelayLength=1  InitialCondition=ee_initial_orientation
  Delay2 : Delay  DelayLength=1  InitialCondition=ee_initial_position
  Gripper input : Subsystem
  Inverse Kinematics : robotmaniplib/Inverse Kinematics  RigidBodyTree=lbr  EndEffector=iiwa_link_ee  ShowInfo=on  SolverName=Levenberg-Marquardt  EnforceJointLimits=on  MaxIterations=1500  MaxTime=10  GradientTolerance=1e-7  SolutionTolerance=1e-6  StepTolerance=1e-14  ErrorChangeTolerance=1e-12  UseErrorDamping=on  DampingBias=0.0025
      settings: SourceProductName=Robotics System Toolbox
  KUKA Gripper : Subsystem
  "KUKA_iiwa 1 " : Subsystem  mask{base_pos=base_initial_position, base_rot=base_initial_orientation}
      mask prompts: base_pos "position [x y z]' (m)"; base_rot "orientation [y p r]' (rad)"
  Reference Frame : sm_lib/Frames and Transforms/Reference Frame
  Rigid Transform : sm_lib/Frames and Transforms/Rigid Transform  TranslationMethod=None  TranslationStandardOffset=0  TranslationLengthUnit=m  TranslationStandardAxis=+Z  TranslationCartesianOffset=[0 0 0]  TranslationROffset=0  TranslationROffsetUnits=m  TranslationZOffset=0  TranslationZOffsetUnits=m  TranslationThetaOffset=0  TranslationThetaOffsetUnits=deg  RotationMethod=RotationSequence  RotationAngleUnits=deg  RotationStandardAxis=+Z  RotationAngle=0.0  RotationArbitraryAxis=[0 0 1]  FollAlignAxisA=+X  BaseAlignAxisA=+Y  FollAlignAxisB=+Y  BaseAlignAxisB=+Z  RotationSequenceAxes=FollowerAxes  RotationSequence=XYZ  RotationSequenceAngles=[-90 -90 0]  RotationSequenceAnglesUnits=deg  RotationMatrix=[1 0 0; 0 1 0; 0 0 1]
  Rigid Transform1 : sm_lib/Frames and Transforms/Rigid Transform  TranslationMethod=Cartesian  TranslationStandardOffset=0  TranslationLengthUnit=cm  TranslationStandardAxis=+Z  TranslationCartesianOffset=[2*beam_radius 0 0]  TranslationROffset=0  TranslationROffsetUnits=m  TranslationZOffset=0  TranslationZOffsetUnits=m  TranslationThetaOffset=0  TranslationThetaOffsetUnits=deg  RotationMethod=RotationSequence  RotationAngleUnits=deg  RotationStandardAxis=+Z  RotationAngle=0.0  RotationArbitraryAxis=[0 0 1]  FollAlignAxisA=+X  BaseAlignAxisA=+Y  FollAlignAxisB=+Y  BaseAlignAxisB=+Z  RotationSequenceAxes=FollowerAxes  RotationSequence=XYZ  RotationSequenceAngles=[0 0 0]  RotationSequenceAnglesUnits=deg  RotationMatrix=[1 0 0; 0 1 0; 0 0 1]
  Terminator : Terminator
  base : PMIOPort  Side=Left
  gripper : PMIOPort  Port=2  Side=Right
  ypr : Outport
  X : Outport  Port=2
  wires:
  Inverse Kinematics/1 -> Delay/1, "KUKA_iiwa 1 "/1(qDesired)  "Conn2"
  Coordinate Transformation Conversion1/1 -> Inverse Kinematics/1
  Constant/1 -> Inverse Kinematics/2
  Inverse Kinematics/2 -> Terminator/1
  "KUKA_iiwa 1 "/1(X) -> Delay2/1
  "KUKA_iiwa 1 "/2(R) -> Coordinate Transformation Conversion/1
  Coordinate Transformation Conversion/1 -> Delay1/1
  ypr_new/1 -> Coordinate Transformation Conversion1/1
  pos_new/1 -> Coordinate Transformation Conversion1/2
  Delay2/1 -> X/1
  Delay1/1 -> ypr/1
  Delay/1 -> Inverse Kinematics/3
  connections:
  base/RConn1 -- "KUKA_iiwa 1 "/LConn1
  KUKA Gripper/LConn1 -- Rigid Transform/RConn1
  Rigid Transform/LConn1 -- "KUKA_iiwa 1 "/RConn1
  gripper/RConn1 -- Rigid Transform1/RConn1
  Rigid Transform1/LConn1 -- KUKA Gripper/RConn1
  KUKA Gripper/LConn2 -- Gripper input/RConn1 -- KUKA Gripper/LConn3
  Gripper input/RConn2 -- KUKA Gripper/LConn4
  "KUKA_iiwa 1 "/LConn2 -- Reference Frame/RConn1

== system alignment_bending_procedure_n_6/Subsystem ==
  beam_state_wf : Inport
  beam_state_wf_des : Inport  Port=2
  J : Inport  Port=3
  xyz_wf_left : Inport  Port=4
  xyz_wf_right : Inport  Port=5
  Constant1 : Constant  Value=fixture_x
  Delay1 : Delay  DelayLength=1  InitialCondition=-9999*ones(5,1)
  Delay2 : Delay  DelayLength=1  InitialCondition=0
  To Workspace : ToWorkspace  VariableName=deformation_state  SampleTime=T
      settings: Save2DSignal=2-D array (concatenate along first dimension)
  To Workspace1 : ToWorkspace  VariableName=deformation_state_des  SampleTime=T
      settings: Save2DSignal=2-D array (concatenate along first dimension)
  To Workspace2 : ToWorkspace  VariableName=beam_state_wf  SampleTime=T
      settings: Save2DSignal=2-D array (concatenate along first dimension)
  deformation ctrl : MATLAB Function  TreatAsAtomicUnit=on
  deformation_input_msr : MATLAB Function  TreatAsAtomicUnit=on
  sampling_time1 : Constant  Value=wf_T_rf_left
  sampling_time2 : Constant  Value=wf_T_rf_right
  deformation_state_des : Outport
  wires:
  deformation ctrl/1(deformation_state_des_new) -> deformation_state_des/1, To Workspace1/1, Delay1/1
  beam_state_wf/1 -> To Workspace2/1, deformation ctrl/1(beam_state_wf)
  beam_state_wf_des/1 -> deformation ctrl/2(beam_state_wf_des)
  xyz_wf_right/1 -> deformation_input_msr/2(xyz_rf_right)
  deformation_input_msr/1(deformation_state) -> deformation ctrl/5(deformation_state), To Workspace/1
  Delay2/1 -> deformation ctrl/7(n_iterations_old)
  deformation ctrl/2(n_iterations_new) -> Delay2/1
  Delay1/1 -> deformation ctrl/6(deformation_state_des_old)
  xyz_wf_left/1 -> deformation_input_msr/1(xyz_rf_left)
  J/1 -> deformation ctrl/3(J)
  sampling_time2/1 -> deformation_input_msr/4(wf_T_rf_right)
  sampling_time1/1 -> deformation_input_msr/3(wf_T_rf_left)
  Constant1/1 -> deformation ctrl/4(x_wf_des)

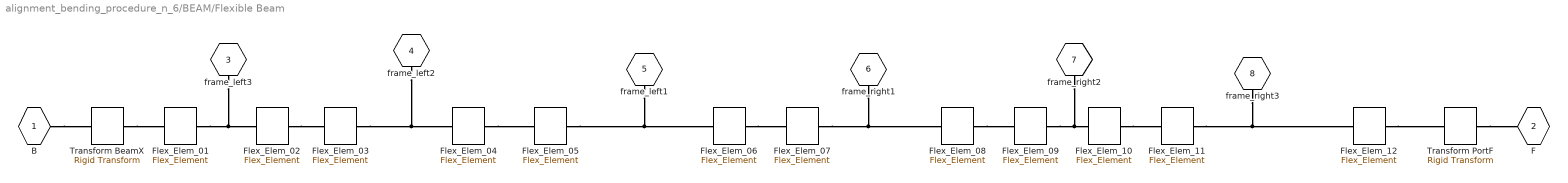
== system alignment_bending_procedure_n_6/BEAM/Flexible Beam ==
  Flex_Elem_01 : sm_flex_body_lib/Lumped Parameter/Bodies/Flex_Element  be_length=elem_length  rho=rho  be_color=beam_color  be_opacity=beam_opacity  krot_beamz_elem=krot_beamz  brot_beamz_elem=brot_beamz  krot_beamy_elem=krot_beamy  brot_beamy_elem=brot_beamy  krot_beamx_elem=krot_beamx  brot_beamx_elem=brot_beamx  ktra_beamx_elem=ktra_beamx  btra_beamx_elem=btra_beamx  radio_flextype_elem=Rotation: Z
  Flex_Elem_02 : sm_flex_body_lib/Lumped Parameter/Bodies/Flex_Element  be_length=elem_length  rho=rho  be_color=beam_color  be_opacity=beam_opacity  krot_beamz_elem=krot_beamz  brot_beamz_elem=brot_beamz  krot_beamy_elem=krot_beamy  brot_beamy_elem=brot_beamy  krot_beamx_elem=krot_beamx  brot_beamx_elem=brot_beamx  ktra_beamx_elem=ktra_beamx  btra_beamx_elem=btra_beamx  radio_flextype_elem=Rotation: Z
  Flex_Elem_03 : sm_flex_body_lib/Lumped Parameter/Bodies/Flex_Element  be_length=elem_length  rho=rho  be_color=beam_color  be_opacity=beam_opacity  krot_beamz_elem=krot_beamz  brot_beamz_elem=brot_beamz  krot_beamy_elem=krot_beamy  brot_beamy_elem=brot_beamy  krot_beamx_elem=krot_beamx  brot_beamx_elem=brot_beamx  ktra_beamx_elem=ktra_beamx  btra_beamx_elem=btra_beamx  radio_flextype_elem=Rotation: Z
  Flex_Elem_04 : sm_flex_body_lib/Lumped Parameter/Bodies/Flex_Element  be_length=elem_length  rho=rho  be_color=beam_color  be_opacity=beam_opacity  krot_beamz_elem=krot_beamz  brot_beamz_elem=brot_beamz  krot_beamy_elem=krot_beamy  brot_beamy_elem=brot_beamy  krot_beamx_elem=krot_beamx  brot_beamx_elem=brot_beamx  ktra_beamx_elem=ktra_beamx  btra_beamx_elem=btra_beamx  radio_flextype_elem=Rotation: Z
  Flex_Elem_05 : sm_flex_body_lib/Lumped Parameter/Bodies/Flex_Element  be_length=elem_length  rho=rho  be_color=beam_color  be_opacity=beam_opacity  krot_beamz_elem=krot_beamz  brot_beamz_elem=brot_beamz  krot_beamy_elem=krot_beamy  brot_beamy_elem=brot_beamy  krot_beamx_elem=krot_beamx  brot_beamx_elem=brot_beamx  ktra_beamx_elem=ktra_beamx  btra_beamx_elem=btra_beamx  radio_flextype_elem=Rotation: Z
  Flex_Elem_06 : sm_flex_body_lib/Lumped Parameter/Bodies/Flex_Element  be_length=elem_length  rho=rho  be_color=beam_color  be_opacity=beam_opacity  krot_beamz_elem=krot_beamz  brot_beamz_elem=brot_beamz  krot_beamy_elem=krot_beamy  brot_beamy_elem=brot_beamy  krot_beamx_elem=krot_beamx  brot_beamx_elem=brot_beamx  ktra_beamx_elem=ktra_beamx  btra_beamx_elem=btra_beamx  radio_flextype_elem=Rotation: Z
  Flex_Elem_07 : sm_flex_body_lib/Lumped Parameter/Bodies/Flex_Element  be_length=elem_length  rho=rho  be_color=beam_color  be_opacity=beam_opacity  krot_beamz_elem=krot_beamz  brot_beamz_elem=brot_beamz  krot_beamy_elem=krot_beamy  brot_beamy_elem=brot_beamy  krot_beamx_elem=krot_beamx  brot_beamx_elem=brot_beamx  ktra_beamx_elem=ktra_beamx  btra_beamx_elem=btra_beamx  radio_flextype_elem=Rotation: Z
  Flex_Elem_08 : sm_flex_body_lib/Lumped Parameter/Bodies/Flex_Element  be_length=elem_length  rho=rho  be_color=beam_color  be_opacity=beam_opacity  krot_beamz_elem=krot_beamz  brot_beamz_elem=brot_beamz  krot_beamy_elem=krot_beamy  brot_beamy_elem=brot_beamy  krot_beamx_elem=krot_beamx  brot_beamx_elem=brot_beamx  ktra_beamx_elem=ktra_beamx  btra_beamx_elem=btra_beamx  radio_flextype_elem=Rotation: Z
  Flex_Elem_09 : sm_flex_body_lib/Lumped Parameter/Bodies/Flex_Element  be_length=elem_length  rho=rho  be_color=beam_color  be_opacity=beam_opacity  krot_beamz_elem=krot_beamz  brot_beamz_elem=brot_beamz  krot_beamy_elem=krot_beamy  brot_beamy_elem=brot_beamy  krot_beamx_elem=krot_beamx  brot_beamx_elem=brot_beamx  ktra_beamx_elem=ktra_beamx  btra_beamx_elem=btra_beamx  radio_flextype_elem=Rotation: Z
  Flex_Elem_10 : sm_flex_body_lib/Lumped Parameter/Bodies/Flex_Element  be_length=elem_length  rho=rho  be_color=beam_color  be_opacity=beam_opacity  krot_beamz_elem=krot_beamz  brot_beamz_elem=brot_beamz  krot_beamy_elem=krot_beamy  brot_beamy_elem=brot_beamy  krot_beamx_elem=krot_beamx  brot_beamx_elem=brot_beamx  ktra_beamx_elem=ktra_beamx  btra_beamx_elem=btra_beamx  radio_flextype_elem=Rotation: Z
  Flex_Elem_11 : sm_flex_body_lib/Lumped Parameter/Bodies/Flex_Element  be_length=elem_length  rho=rho  be_color=beam_color  be_opacity=beam_opacity  krot_beamz_elem=krot_beamz  brot_beamz_elem=brot_beamz  krot_beamy_elem=krot_beamy  brot_beamy_elem=brot_beamy  krot_beamx_elem=krot_beamx  brot_beamx_elem=brot_beamx  ktra_beamx_elem=ktra_beamx  btra_beamx_elem=btra_beamx  radio_flextype_elem=Rotation: Z
  Flex_Elem_12 : sm_flex_body_lib/Lumped Parameter/Bodies/Flex_Element  be_length=elem_length  rho=rho  be_color=beam_color  be_opacity=beam_opacity  krot_beamz_elem=krot_beamz  brot_beamz_elem=brot_beamz  krot_beamy_elem=krot_beamy  brot_beamy_elem=brot_beamy  krot_beamx_elem=krot_beamx  brot_beamx_elem=brot_beamx  ktra_beamx_elem=ktra_beamx  btra_beamx_elem=btra_beamx  radio_flextype_elem=Rotation: Z
  Transform BeamX : sm_lib/Frames and Transforms/Rigid Transform  TranslationMethod=StandardAxis  TranslationStandardOffset=0  TranslationLengthUnit=m  TranslationStandardAxis=+Z  TranslationCartesianOffset=[0 0 0]  TranslationROffset=0  TranslationROffsetUnits=m  TranslationZOffset=0  TranslationZOffsetUnits=m  TranslationThetaOffset=0  TranslationThetaOffsetUnits=deg  RotationMethod=StandardAxis  RotationAngleUnits=deg  RotationStandardAxis=+Y  RotationAngle=90  RotationArbitraryAxis=[0 0 1]  FollAlignAxisA=+X  BaseAlignAxisA=+Y  FollAlignAxisB=+Y  BaseAlignAxisB=+Z  RotationSequenceAxes=FollowerAxes  RotationSequence=XYX  RotationSequenceAngles=[0 0 0]  RotationSequenceAnglesUnits=deg  RotationMatrix=[1 0 0; 0 1 0; 0 0 1]
  Transform PortF : sm_lib/Frames and Transforms/Rigid Transform  TranslationMethod=None  TranslationStandardOffset=0  TranslationLengthUnit=m  TranslationStandardAxis=+Z  TranslationCartesianOffset=[0 0 0]  TranslationROffset=0  TranslationROffsetUnits=m  TranslationZOffset=0  TranslationZOffsetUnits=m  TranslationThetaOffset=0  TranslationThetaOffsetUnits=deg  RotationMethod=StandardAxis  RotationAngleUnits=deg  RotationStandardAxis=+Y  RotationAngle=-90  RotationArbitraryAxis=[0 0 1]  FollAlignAxisA=+X  BaseAlignAxisA=+Y  FollAlignAxisB=+Y  BaseAlignAxisB=+Z  RotationSequenceAxes=FollowerAxes  RotationSequence=XYX  RotationSequenceAngles=[0 0 0]  RotationSequenceAnglesUnits=deg  RotationMatrix=[1 0 0; 0 1 0; 0 0 1]
  B : PMIOPort  Side=Left
  F : PMIOPort  Port=2  Side=Right
  frame_left3 : PMIOPort  Port=3  Side=Right
  frame_left2 : PMIOPort  Port=4  Side=Right
  frame_left1 : PMIOPort  Port=5  Side=Right
  frame_right1 : PMIOPort  Port=6  Side=Right
  frame_right2 : PMIOPort  Port=7  Side=Right
  frame_right3 : PMIOPort  Port=8  Side=Right
  connections:
  B/RConn1 -- Transform BeamX/LConn1
  Transform BeamX/RConn1 -- Flex_Elem_01/LConn1
  Flex_Elem_01/RConn1 -- frame_left3/RConn1 -- Flex_Elem_02/LConn1
  Flex_Elem_02/RConn1 -- Flex_Elem_03/LConn1
  Flex_Elem_03/RConn1 -- frame_left2/RConn1 -- Flex_Elem_04/LConn1
  Flex_Elem_04/RConn1 -- Flex_Elem_05/LConn1
  Flex_Elem_05/RConn1 -- frame_left1/RConn1 -- Flex_Elem_06/LConn1
  Flex_Elem_06/RConn1 -- Flex_Elem_07/LConn1
  Flex_Elem_07/RConn1 -- frame_right1/RConn1 -- Flex_Elem_08/LConn1
  Flex_Elem_08/RConn1 -- Flex_Elem_09/LConn1
  Flex_Elem_09/RConn1 -- frame_right2/RConn1 -- Flex_Elem_10/LConn1
  Flex_Elem_10/RConn1 -- Flex_Elem_11/LConn1
  Flex_Elem_11/RConn1 -- Flex_Elem_12/LConn1 -- frame_right3/RConn1
  Flex_Elem_12/RConn1 -- Transform PortF/LConn1
  Transform PortF/RConn1 -- F/RConn1

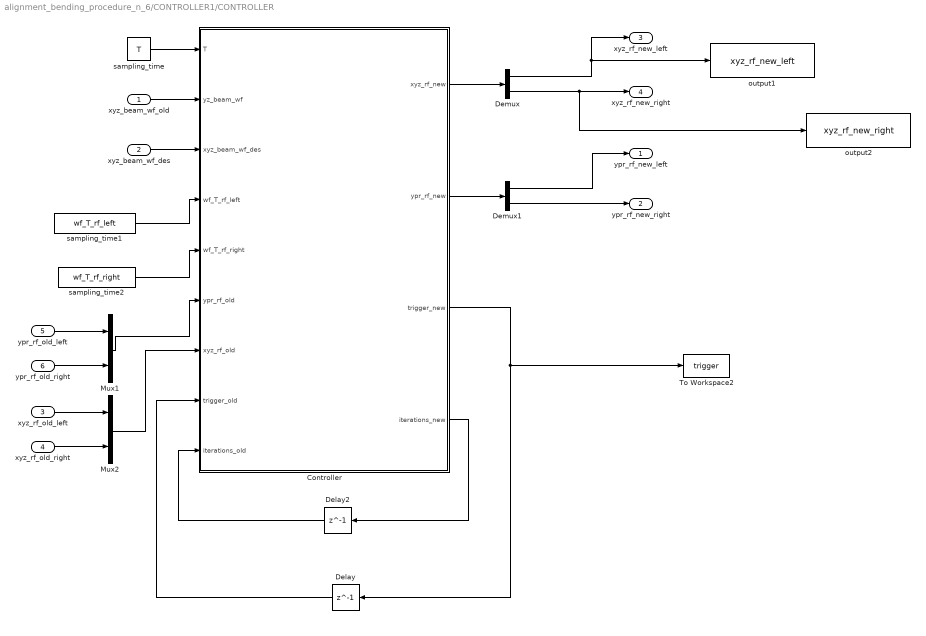
== system alignment_bending_procedure_n_6/CONTROLLER1/CONTROLLER ==
  xyz_beam_wf_old : Inport
  xyz_beam_wf_des : Inport  Port=2
  "xyz_rf_old_left " : Inport  Port=3
  xyz_rf_old_right : Inport  Port=4
  ypr_rf_old_left : Inport  Port=5
  ypr_rf_old_right : Inport  Port=6
  Controller : MATLAB Function  TreatAsAtomicUnit=on
  Delay : Delay  DelayLength=1  InitialCondition=zeros(5,1)
  Delay2 : Delay  DelayLength=1  InitialCondition=0  SampleTime=T
  Demux : Demux  Outputs=[3 3]
  Demux1 : Demux  Outputs=[3 3]
  Mux1 : Mux  Inputs=2
  Mux2 : Mux  Inputs=2
  To Workspace2 : ToWorkspace  VariableName=trigger  SampleTime=-1
  output1 : ToWorkspace  VariableName=xyz_rf_new_left  SampleTime=-1
      settings: Save2DSignal=2-D array (concatenate along first dimension)
  output2 : ToWorkspace  VariableName=xyz_rf_new_right  SampleTime=-1
      settings: Save2DSignal=2-D array (concatenate along first dimension)
  sampling_time : Constant  Value=T
  sampling_time1 : Constant  Value=wf_T_rf_left
  sampling_time2 : Constant  Value=wf_T_rf_right
  ypr_rf_new_left : Outport
  ypr_rf_new_right : Outport  Port=2
  xyz_rf_new_left : Outport  Port=3
  xyz_rf_new_right : Outport  Port=4
  wires:
  Delay/1 -> Controller/8(trigger_old)
  Controller/3(trigger_new) -> Delay/1, To Workspace2/1
  sampling_time/1 -> Controller/1(T)
  xyz_beam_wf_old/1 -> Controller/2(yz_beam_wf)
  ypr_rf_old_left/1 -> Mux1/1
  ypr_rf_old_right/1 -> Mux1/2
  "xyz_rf_old_left "/1 -> Mux2/1
  xyz_rf_old_right/1 -> Mux2/2
  Controller/1(xyz_rf_new) -> Demux/1
  Controller/2(ypr_rf_new) -> Demux1/1
  xyz_beam_wf_des/1 -> Controller/3(xyz_beam_wf_des)
  Mux1/1 -> Controller/6(ypr_rf_old)
  Mux2/1 -> Controller/7(xyz_rf_old)
  Demux/1 -> output1/1, xyz_rf_new_left/1
  Demux1/1 -> ypr_rf_new_left/1
  Demux1/2 -> ypr_rf_new_right/1
  sampling_time1/1 -> Controller/4(wf_T_rf_left)
  sampling_time2/1 -> Controller/5(wf_T_rf_right)
  Demux/2 -> output2/1, xyz_rf_new_right/1
  Delay2/1 -> Controller/9(iterations_old)
  Controller/4(iterations_new) -> Delay2/1
